simulink model "Ex1_Arithmetic_operations"  (Simulink 8.9)
settings: Solver=VariableStepAuto  StartTime=0.0  StopTime=10.0  RelTol=1e-3
settings Model: Creator=sulaymon.eshkabilov  LastModifiedBy=sulaymon.eshkabilov
settings DataIOCC: LimitDataPoints=off  SaveFormat=Dataset  SignalLoggingSaveFormat=Dataset
settings OptimizationCC: LifeSpan=auto
settings DebuggingCC: UnderspecifiedInitializationDetection=Simplified  MergeDetectMultiDrivingBlocksExec=error  FcnCallInpInsideContextMsg=error  StateNameClashWarn=none  SFUnexpectedBacktrackingDiag=error  SFNoUnconditionalDefaultTransitionDiag=error  SFExecutionAtInitializationDiag=warning
settings HardwareCC: ProdBitPerPointer=64  ProdBitPerSizeT=64  ProdBitPerPtrDiffT=64  ProdLargestAtomicFloat=Float  ProdIntDivRoundTo=Zero  ProdEndianess=LittleEndian  ProdWordSize=64  ProdHWDeviceType=Intel->x86-64 (Windows64)
settings ModelReferenceCC: PropagateSignalLabelsOutOfModel=on
settings GRTTargetCC: TargetLangStandard=C99 (ISO)  GeneratePreprocessorConditionals=Use local settings  CombineOutputUpdateFcns=on  GRTInterface=off
settings ConfigComp: CovMetricSettings=dwe  CovHtmlReporting=off  CovSaveCumulativeToWorkspaceVar=off  CovSaveSingleToWorkspaceVar=off  CovExternalEMLEnable=on

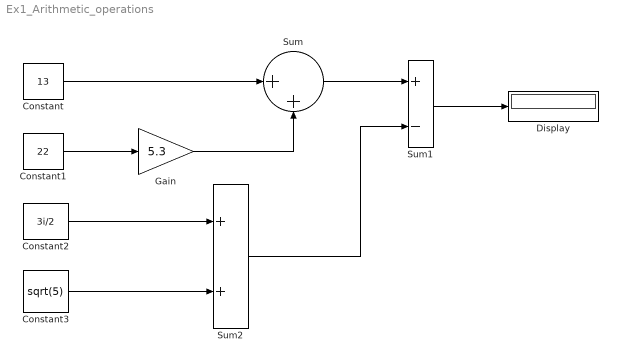
== system Ex1_Arithmetic_operations ==
  Constant : Constant  Value=13
  Constant1 : Constant  Value=22
  Constant2 : Constant  Value=3i/2
  Constant3 : Constant  Value=sqrt(5)
  Display : Display
  Gain : Gain  Gain=5.3
  Sum : Sum  Inputs=|++
  Sum1 : Sum  Inputs=+-
  Sum2 : Sum
  wires:
  Constant1/1 -> Gain/1
  Gain/1 -> Sum/2
  Constant/1 -> Sum/1
  Constant2/1 -> Sum2/1
  Constant3/1 -> Sum2/2
  Sum/1 -> Sum1/1
  Sum2/1 -> Sum1/2
  Sum1/1 -> Display/1
